simulink model "pid_control_V1"  (R2025b)
settings: Solver=FixedStepAuto  StartTime=0.0  StopTime=tsim  FixedStep=0.01  RelTol=1e-3
undefined symbols (not defined in the file): Cp, F, h_sp, Kd_h, Kd_pitch, Ki_h, Ki_pitch, Kp_h, Kp_pitch, Light, MIL, state, theta_sp, Tp, u_nom, x0
libraries: aerolibactuator x5, ros2lib x2, slpidlib x2, robotcorelib x1, aerolibwind2 x1
settings Model: Creator=sofij  LastModifiedBy=facyu
settings SolverCC: AlgebraicLoopSolver=TrustRegion
settings OptimizationCC: DefaultParameterBehavior=Inlined  EnhancedBackFolding=on  PassReuseOutputArgsAs=Individual arguments  ZeroExternalMemoryAtStartup=off  ZeroInternalMemoryAtStartup=off  MaxStackSize=64  OptimizeBlockOrder=speed  DifferentSizesBufferReuse=on  OptimizationCustomize=off  EfficientTunableParamExpr=on
settings DebuggingCC: ParameterTunabilityLossMsg=error  UnconnectedInputMsg=warning  UnconnectedOutputMsg=warning  UnconnectedLineMsg=warning  SFUnexpectedBacktrackingDiag=warning  SFNoUnconditionalDefaultTransitionDiag=warning
settings HardwareCC: ProdBitPerLong=64.0  ProdHWDeviceType=Intel->x86-64 (Linux 64)  UseEmbeddedCoderFeatures=off
settings ModelReferenceCC: EnableRefExpFcnMdlSchedulingChecks=on
settings SFSimCC: MATLABDynamicMemAlloc=off
settings RTWCC: SystemTargetFile=ert.tlc  HardwareBoard=Robot Operating System 2 (ROS 2)  TLCOptions="-aInlineSetEventsForThisBaseRateFcn=TLC_FALSE -aSuppressMultiTaskScheduler=TLC_FALSE  -aRateBasedStepFcn=0"  TemplateMakefile=ert_default_tmf  GenerateReport=on  Toolchain=Colcon Tools  BuildConfiguration=Debug  LaunchReport=on  TargetLang=C++  GPUComputeCapability=3.5  DLArmComputeVersion=19.05  Description=Embedded Coder
settings CodeAppCC: ForceParamTrailComments=on  IgnoreCustomStorageClasses=off  OperatorAnnotations=on  SimulinkDataObjDesc=on  SFDataObjDesc=on  InsertBlockDesc=on  EnableCustomComments=on
settings ERTTargetCC: ExtModeTransport=2.0  ExtModeStaticAlloc=on  ExtModeAutomaticAllocSize=off  ExtModeMexFile=ext_xcp  ExtModeIntrfLevel=Level2 - Open  RootIOFormat=Structure reference  CodeInterfacePackaging=C++ class  SupportNonInlinedSFcns=on

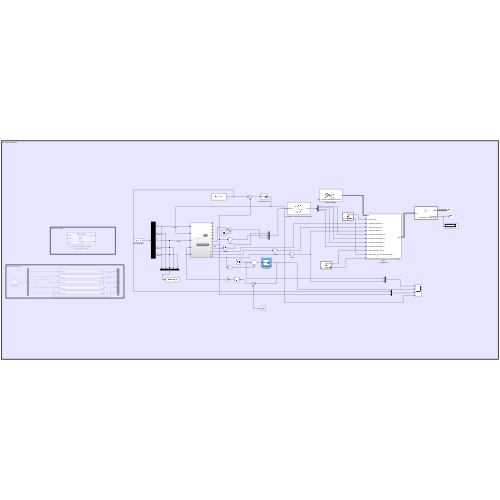
[thumbnail: Simulink's stored preview of the top-level diagram]
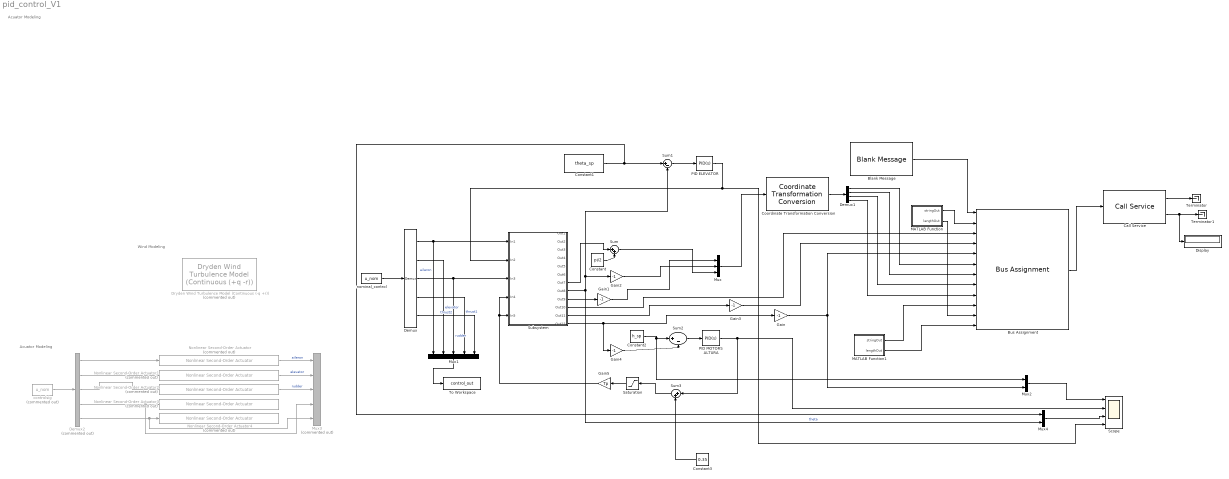
== system pid_control_V1 ==
  note: Wind Modeling
  note: Acuator Modeling
  note: Acuator Modeling
  Blank Message : ros2lib/Blank Message  messageClass=Service Request  entityType=gazebo_msgs/SetEntityState  messageType=gazebo_msgs/SetEntityStateRequest  SampleTime=0.01
  Bus Assignment : BusAssignment  AssignedSignals=state.name,state.pose.position.x,state.pose.position.y,state.pose.position.z,state.pose.orientation.w,state.pose.orientation.z,state.pose.orientation.y,state.pose.orientation.x,state.reference_frame,state.name_SL_Info.CurrentLength,state.reference_frame_SL_Info.CurrentLength
  Call Service : ros2lib/Call Service  topicSource=Specify your own  service=/gazebo/set_entity_state  serviceType=gazebo_msgs/SetEntityState  connectionTimeout=5  ShowErrorCodeOutput=on  legacyBusStruct=off  QOSHistory=Keep last  QOSDepth=1  QOSReliability=Reliable  QOSDurability=Volatile  QOSDeadline=Inf  QOSLifespan=Inf  QOSLiveliness=Automatic  QOSLeaseDuration=Inf  QOSAvoidROSNamespaceConventions=off
  Constant : Constant  Value=pi/2
  Constant1 : Constant  Value=theta_sp
  Constant2 : Constant  Value=h_sp
  Constant3 : Constant  Value=0.35
  Coordinate Transformation Conversion : robotcorelib/Coordinate Transformation Conversion  InputRepresentation=Euler Angles  InputEulerSequence=ZYX  ShowTrVecInputPort=on  OutputRepresentation=Quaternion  OutputEulerSequence=ZYX  ShowTrVecOutputPort=on  SimulateUsing=Interpreted execution
      settings: LibrarySourceBlock=roslib/Utilities/Coordinate Transformation Conversion
  Demux : Demux  Outputs=5
  Demux1 : Demux
  Demux2 : Demux  Commented=on  Outputs=5
  Display : Display
  Dryden Wind Turbulence Model (Continuous (-q +r)) : aerolibwind2/Dryden Wind Turbulence Model  (Continuous (+q -r))  Commented=on  units=Metric (MKS)  spec=MIL-F-8785C  model=Continuous Dryden (-q +r)  W20=15  Wdeg=0  TurbProb=10^-2 - Light  L_high=533.4  Wingspan=10  ts=0.1  Seed=[23341 23342 23343 23344]  T_on=on
  Gain{,1..4} (5 alike) : Gain  Gain=-1
  Gain5 : Gain  Gain=Tp
  MATLAB Function : MATLAB Function  TreatAsAtomicUnit=on
  MATLAB Function1 : MATLAB Function  TreatAsAtomicUnit=on
  Mux : Mux  Inputs=3
  Mux1 : Mux  Inputs=5
  Mux2 : Mux  Inputs=2
  Mux3 : Mux  Commented=on  Inputs=5
  Mux4 : Mux  Inputs=2
  Nonlinear Second-Order Actuator : aerolibactuator/Nonlinear Second-Order Actuator  Commented=on  wn_fin=1  z_fin=0.3  fin_max=15*pi/180  fin_min=-20*pi/180  fin_maxrate=500*pi/180  fin_act_0=0  fin_act_vel=0
  Nonlinear Second-Order Actuator1 : aerolibactuator/Nonlinear Second-Order Actuator  Commented=on  wn_fin=1  z_fin=0.3  fin_max=20*pi/180  fin_min=-20*pi/180  fin_maxrate=500*pi/180  fin_act_0=0  fin_act_vel=0
  Nonlinear Second-Order Actuator2 : aerolibactuator/Nonlinear Second-Order Actuator  Commented=on  wn_fin=1  z_fin=0.3  fin_max=15*pi/180  fin_min=-15*pi/180  fin_maxrate=500*pi/180  fin_act_0=0  fin_act_vel=0
  Nonlinear Second-Order Actuator3 : aerolibactuator/Nonlinear Second-Order Actuator  Commented=on  wn_fin=1  z_fin=0.3  fin_max=100  fin_min=0  fin_maxrate=500*pi/180  fin_act_0=0  fin_act_vel=0
  Nonlinear Second-Order Actuator4 : aerolibactuator/Nonlinear Second-Order Actuator  Commented=on  wn_fin=1  z_fin=0.3  fin_max=100  fin_min=0  fin_maxrate=500*pi/180  fin_act_0=0  fin_act_vel=0
  PID ELEVATOR : slpidlib/PID Controller  Controller=PID  Form=Parallel  TimeDomain=Continuous-time  UseExternalTs=off  SampleTime=-1  IntegratorMethod=Forward Euler  FilterMethod=Forward Euler  ControllerParametersSource=internal  P=Kp_pitch  I=Ki_pitch  UseKiTs=off  D=Kd_pitch  UseExternalDerivativeSource=off  N=100  UseFilter=on  TunerSelectOption=Transfer Function Based (PID Tuner App)  InitialConditionSource=internal  InitialConditionForIntegrator=0  InitialConditionForFilter=0  DifferentiatorICPrevScaledInput=0  ExternalReset=none  TrackingMode=off  Kt=1  LimitOutput=on  SatLimitsSource=internal  UpperSaturationLimit=20*pi/180  LowerSaturationLimit=-20*pi/180  LinearizeAsGain=on  AntiWindupMode=clamping  Kb=1  LimitIntegrator=off  UpperIntegratorSaturationLimit=inf  LowerIntegratorSaturationLimit=-inf  POutMin=[]  POutMax=[]  IOutMin=[]  IOutMax=[]  DOutMin=[]  DOutMax=[]  NOutMin=[]  NOutMax=[]  SumOutMin=[]  SumOutMax=[]  SaturationOutMin=[]  SaturationOutMax=[]  PParamMin=[]  PParamMax=[]  IParamMin=[]  IParamMax=[]  DParamMin=[]  DParamMax=[]  NParamMin=[]  NParamMax=[]  KbParamMin=[]  KbParamMax=[]  KtParamMin=[]  KtParamMax=[]  KbOutMin=[]  KbOutMax=[]  KtOutMin=[]  KtOutMax=[]  IntegratorOutMin=[]  IntegratorOutMax=[]  FilterOutMin=[]  FilterOutMax=[]  SumI1OutMin=[]  SumI1OutMax=[]  SumI2OutMin=[]  SumI2OutMax=[]  SumI3OutMin=[]  SumI3OutMax=[]  SumI4OutMin=[]  SumI4OutMax=[]  SumDOutMin=[]  SumDOutMax=[]  DifferentiatorOutMin=[]  DifferentiatorOutMax=[]  FilterDiffOutCoefMin=[]  FilterDiffOutCoefMax=[]  ReciprocalOutMin=[]  ReciprocalOutMax=[]  SumDenOutMin=[]  SumDenOutMax=[]  SumNumOutMin=[]  SumNumOutMax=[]  DivideOutMin=[]  DivideOutMax=[]  UdiffTsProdOutMin=[]  UdiffTsProdOutMax=[]  NTsProdOutMin=[]  NTsProdOutMax=[]  UintegralTsProdOutMin=[]  UintegralTsProdOutMax=[]  UngainTsProdOutMin=[]  UngainTsProdOutMax=[]  ClampingZeroOutDataTypeStr=Inherit: Inherit via back propagation  ClampingZeroOutMin=[]  ClampingZeroOutMax=[]  FilterDenConstantOutDataTypeStr=Inherit: Inherit via back propagation  FilterDenConstantOutMin=[]  FilterDenConstantOutMax=[]  PCopyOutDataTypeStr=Inherit: Inherit via back propagation  PCopyOutMin=[]  PCopyOutMax=[]  NCopyOutDataTypeStr=Inherit: Inherit via back propagation  NCopyOutMin=[]  NCopyOutMax=[]  IntegratorContinuousStateAttributes=''  IntegratorStateMustResolveToSignalObject=off  IntegratorRTWStateStorageClass=Auto  FilterContinuousStateAttributes=''  FilterStateMustResolveToSignalObject=off  FilterRTWStateStorageClass=Auto  ParallelPVariant=InternalParameters  IdealPVariant=Disabled  IVariant=InternalParameters  DVariant=InternalParameters  IntegratorVariant=Continuous  SatVariant=Enabled  AWVariant=ContClampingParallel  PCopyVariant=Disabled  TRVariant=Disabled  FdbkBlocksVariant=Forward  IdealPFdbkVariant=Disabled  SatFdbkVariant=Disabled  DerivativeFilterVariant=ContFilter  NVariant=InternalParameters  NCopyVariant=Disabled  FilterICVariant=InternalICsFilter  IntegratorICVariant=InternalICs  ExternalResetVariant=Disabled  TRSumVariant=Passthrough  SumFdbkVariant=Disabled  SumVariant=Sum_PID  TsampFilterVariant=InternalTs  TsampNgainVariant=Passthrough  TsampIntegralVariant=Disabled_SignalSpec  ExternalSaturationOutDataTypeStr=Inherit: Same as second input  DerivativeSourceVariant=ErrorSignal  PreIntVariant=InternalPreInt
  PID MOTORS ALTURA : slpidlib/PID Controller  Controller=PID  Form=Parallel  TimeDomain=Continuous-time  UseExternalTs=off  SampleTime=-1  IntegratorMethod=Forward Euler  FilterMethod=Forward Euler  ControllerParametersSource=internal  P=Kp_h  I=Ki_h  UseKiTs=off  D=Kd_h  UseExternalDerivativeSource=off  N=100  UseFilter=on  TunerSelectOption=Transfer Function Based (PID Tuner App)  InitialConditionSource=internal  InitialConditionForIntegrator=0.3  InitialConditionForFilter=0  DifferentiatorICPrevScaledInput=0  ExternalReset=none  TrackingMode=off  Kt=1  LimitOutput=on  SatLimitsSource=internal  UpperSaturationLimit=1  LowerSaturationLimit=0  LinearizeAsGain=on  AntiWindupMode=clamping  Kb=1  LimitIntegrator=off  UpperIntegratorSaturationLimit=inf  LowerIntegratorSaturationLimit=-inf  POutMin=[]  POutMax=[]  IOutMin=[]  IOutMax=[]  DOutMin=[]  DOutMax=[]  NOutMin=[]  NOutMax=[]  SumOutMin=[]  SumOutMax=[]  SaturationOutMin=[]  SaturationOutMax=[]  PParamMin=[]  PParamMax=[]  IParamMin=[]  IParamMax=[]  DParamMin=[]  DParamMax=[]  NParamMin=[]  NParamMax=[]  KbParamMin=[]  KbParamMax=[]  KtParamMin=[]  KtParamMax=[]  KbOutMin=[]  KbOutMax=[]  KtOutMin=[]  KtOutMax=[]  IntegratorOutMin=[]  IntegratorOutMax=[]  FilterOutMin=[]  FilterOutMax=[]  SumI1OutMin=[]  SumI1OutMax=[]  SumI2OutMin=[]  SumI2OutMax=[]  SumI3OutMin=[]  SumI3OutMax=[]  SumI4OutMin=[]  SumI4OutMax=[]  SumDOutMin=[]  SumDOutMax=[]  DifferentiatorOutMin=[]  DifferentiatorOutMax=[]  FilterDiffOutCoefMin=[]  FilterDiffOutCoefMax=[]  ReciprocalOutMin=[]  ReciprocalOutMax=[]  SumDenOutMin=[]  SumDenOutMax=[]  SumNumOutMin=[]  SumNumOutMax=[]  DivideOutMin=[]  DivideOutMax=[]  UdiffTsProdOutMin=[]  UdiffTsProdOutMax=[]  NTsProdOutMin=[]  NTsProdOutMax=[]  UintegralTsProdOutMin=[]  UintegralTsProdOutMax=[]  UngainTsProdOutMin=[]  UngainTsProdOutMax=[]  ClampingZeroOutDataTypeStr=Inherit: Inherit via back propagation  ClampingZeroOutMin=[]  ClampingZeroOutMax=[]  FilterDenConstantOutDataTypeStr=Inherit: Inherit via back propagation  FilterDenConstantOutMin=[]  FilterDenConstantOutMax=[]  PCopyOutDataTypeStr=Inherit: Inherit via back propagation  PCopyOutMin=[]  PCopyOutMax=[]  NCopyOutDataTypeStr=Inherit: Inherit via back propagation  NCopyOutMin=[]  NCopyOutMax=[]  IntegratorContinuousStateAttributes=''  IntegratorStateMustResolveToSignalObject=off  IntegratorRTWStateStorageClass=Auto  FilterContinuousStateAttributes=''  FilterStateMustResolveToSignalObject=off  FilterRTWStateStorageClass=Auto  ParallelPVariant=InternalParameters  IdealPVariant=Disabled  IVariant=InternalParameters  DVariant=InternalParameters  IntegratorVariant=Continuous  SatVariant=Enabled  AWVariant=ContClampingParallel  PCopyVariant=Disabled  TRVariant=Disabled  FdbkBlocksVariant=Forward  IdealPFdbkVariant=Disabled  SatFdbkVariant=Disabled  DerivativeFilterVariant=ContFilter  NVariant=InternalParameters  NCopyVariant=Disabled  FilterICVariant=InternalICsFilter  IntegratorICVariant=InternalICs  ExternalResetVariant=Disabled  TRSumVariant=Passthrough  SumFdbkVariant=Disabled  SumVariant=Sum_PID  TsampFilterVariant=InternalTs  TsampNgainVariant=Passthrough  TsampIntegralVariant=Disabled_SignalSpec  ExternalSaturationOutDataTypeStr=Inherit: Same as second input  DerivativeSourceVariant=ErrorSignal  PreIntVariant=InternalPreInt
  Saturation : Saturate  UpperLimit=1.0  LowerLimit=0.3
  Scope : Scope  NumInputPorts=4
      settings: ActiveDisplayYMinimum=-1.7310534077448412  ActiveDisplayYMaximum=4.7021232527921839  DataLoggingVariableName=ScopeData4
  Subsystem : Subsystem
  Sum : Sum  Inputs=|++
  Sum1 : Sum  Inputs=|+-
  Sum2 : Sum  Inputs=|+-
  Sum3 : Sum  Inputs=|++
  Terminator : Terminator
  Terminator1 : Terminator
  To Workspace : ToWorkspace  VariableName=control_out  SampleTime=-1
      settings: Save2DSignal=2-D array (concatenate along first dimension)
  controlsig : Constant  Commented=on  Value=u_nom
  nominal_control : Constant  Value=u_nom
  wires:
  controlsig/1 -> Demux2/1
  Nonlinear Second-Order Actuator/1 -> Mux3/1  "aileron"
  Demux2/1 -> Nonlinear Second-Order Actuator/1
  Demux2/5 -> Mux3/5, Nonlinear Second-Order Actuator4/1
  Demux2/4 -> Mux3/4, Nonlinear Second-Order Actuator3/1
  Demux2/3 -> Nonlinear Second-Order Actuator2/1
  Demux2/2 -> Nonlinear Second-Order Actuator1/1
  Nonlinear Second-Order Actuator2/1 -> Mux3/3  "rudder"
  Nonlinear Second-Order Actuator1/1 -> Mux3/2  "elevator"
  Demux/3 -> Mux1/3, Subsystem/3(In3)  "rudder"
  nominal_control/1 -> Demux/1
  Demux/1 -> Subsystem/1(In1), Mux1/1  "aileron"
  Blank Message/1 -> Bus Assignment/1
  Subsystem/10(Out10) -> Bus Assignment/3
  Subsystem/11(Out11) -> Gain3/1
  Subsystem/12(Out12) -> Gain4/1, Gain/1
  Subsystem/8(Out8) -> Mux4/2, Gain2/1, Sum1/2  "theta"
  Subsystem/9(Out9) -> Gain1/1
  Mux/1 -> Coordinate Transformation Conversion/1
  Coordinate Transformation Conversion/1 -> Demux1/1
  Demux1/1 -> Bus Assignment/6
  Demux1/2 -> Bus Assignment/7
  Demux1/3 -> Bus Assignment/8
  Demux1/4 -> Bus Assignment/9
  Bus Assignment/1 -> Call Service/1
  Gain/1 -> Mux2/2, Bus Assignment/5
  Call Service/1 -> Terminator/1
  Call Service/2 -> Display/1, Terminator1/1
  MATLAB Function/1(stringOut) -> Bus Assignment/2
  MATLAB Function1/1(stringOut) -> Bus Assignment/10
  MATLAB Function/2(lengthOut) -> Bus Assignment/11
  MATLAB Function1/2(lengthOut) -> Bus Assignment/12
  Gain2/1 -> Mux/2
  Subsystem/7(Out7) -> Sum/1
  Gain3/1 -> Bus Assignment/4
  Gain1/1 -> Mux/1
  Sum/1 -> Mux/3
  Constant/1 -> Sum/2
  Constant1/1 -> Sum1/1, Mux4/1
  Sum1/1 -> PID ELEVATOR/1
  PID ELEVATOR/1 -> Scope/4, Subsystem/2(In2)
  Constant2/1 -> Mux2/1, Sum2/1
  Gain4/1 -> Sum2/2
  Sum2/1 -> PID MOTORS ALTURA/1
  PID MOTORS ALTURA/1 -> Sum3/1, Scope/2
  Mux2/1 -> Scope/1
  Mux4/1 -> Scope/3
  Gain5/1 -> Subsystem/5(In5), Subsystem/4(In4)
  Mux1/1 -> To Workspace/1
  Demux/2 -> Mux1/2  "elevator"
  Demux/4 -> Mux1/4  "thrust1"
  Demux/5 -> Mux1/5  "thrust2"
  Constant3/1 -> Sum3/2
  Saturation/1 -> Gain5/1
  Sum3/1 -> Saturation/1

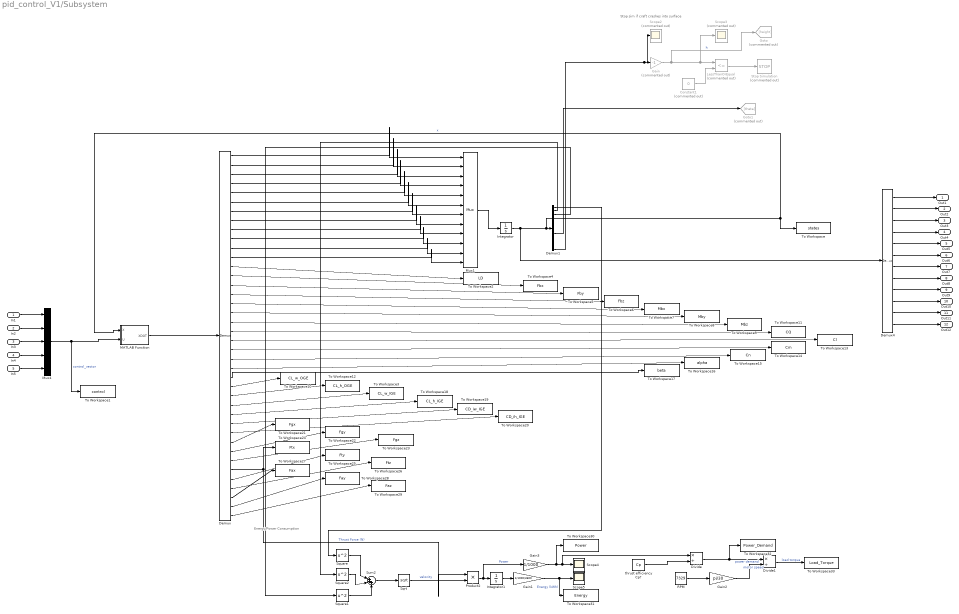
== system pid_control_V1/Subsystem ==
  note: Stop sim if craft crashes into surface
  note: Energy/Power Consumption
  In1 : Inport
  In2 : Inport  Port=2
  In3 : Inport  Port=3
  In4 : Inport  Port=4
  In5 : Inport  Port=5
  Constant1 : Constant  Commented=on  Value=0
  Demux : Demux  Outputs=40
  Demux1 : Demux  Outputs=12
  Demux4 : Demux  Outputs=12
  Divide : Product  Inputs=*/
  Divide1 : Product  Inputs=*/
  Gain : Gain  Commented=on  Gain=-1
  Gain1 : Gain  Gain=1/1000/3600
  Gain2 : Gain  Gain=pi/30
  Gain3 : Gain  Gain=1/1000
  Goto : Goto  Commented=on  GotoTag=height
  Goto1 : Goto  Commented=on  GotoTag=theta
  Integrator : Integrator  InitialCondition=x0
  Integrator1 : Integrator
  LessThanOrEqual : RelationalOperator  Commented=on  Operator=<=  OutDataTypeStr=boolean  RndMeth=Simplest  InputSameDT=off
  MATLAB Function : MATLAB Function  TreatAsAtomicUnit=on
  Mux1 : Mux  Inputs=12
  Mux4 : Mux  Inputs=5
  Product2 : Product
  RPM : Constant  Value=7329
  Scope2 : Scope  Commented=on
      settings: ActiveDisplayYMinimum=-1.36989  ActiveDisplayYMaximum=0.16067
  Scope3 : Scope  Commented=on
      settings: ActiveDisplayYMinimum=-0.16067  ActiveDisplayYMaximum=1.36989  DataLoggingVariableName=ScopeData2
  Scope4 : Scope
      settings: ActiveDisplayYMinimum=-1  ActiveDisplayYMaximum=1  DataLoggingVariableName=ScopeData3
  Scope5 : Scope
  Sqrt : Sqrt
  Square : Math  Operator=square
  Square1 : Math  Operator=square
  Square2 : Math  Operator=square
  Stop Simulation : Stop  Commented=on
  Sum2 : Sum  Inputs=|+++
  To Workspace : ToWorkspace  VariableName=states  SampleTime=-1
  To Workspace1 : ToWorkspace  VariableName=control  SampleTime=-1
  To Workspace10 : ToWorkspace  VariableName=CL_w_OGE  SampleTime=-1
      settings: Save2DSignal=2-D array (concatenate along first dimension)
  To Workspace11 : ToWorkspace  VariableName=CQ  SampleTime=-1
      settings: Save2DSignal=2-D array (concatenate along first dimension)
  To Workspace12 : ToWorkspace  VariableName=CL_h_OGE  SampleTime=-1
      settings: Save2DSignal=2-D array (concatenate along first dimension)
  To Workspace13 : ToWorkspace  VariableName=Cl  SampleTime=-1
      settings: Save2DSignal=2-D array (concatenate along first dimension)
  To Workspace14 : ToWorkspace  VariableName=Cm  SampleTime=-1
      settings: Save2DSignal=2-D array (concatenate along first dimension)
  To Workspace15 : ToWorkspace  VariableName=Cn  SampleTime=-1
      settings: Save2DSignal=2-D array (concatenate along first dimension)
  To Workspace16 : ToWorkspace  VariableName=alpha  SampleTime=-1
      settings: Save2DSignal=2-D array (concatenate along first dimension)
  To Workspace17 : ToWorkspace  VariableName=beta  SampleTime=-1
      settings: Save2DSignal=2-D array (concatenate along first dimension)
  To Workspace18 : ToWorkspace  VariableName=CL_h_IGE  SampleTime=-1
      settings: Save2DSignal=2-D array (concatenate along first dimension)
  To Workspace19 : ToWorkspace  VariableName=CD_iw_IGE  SampleTime=-1
      settings: Save2DSignal=2-D array (concatenate along first dimension)
  To Workspace2 : ToWorkspace  VariableName=LD  SampleTime=-1
      settings: Save2DSignal=2-D array (concatenate along first dimension)
  To Workspace20 : ToWorkspace  VariableName=CD_ih_IGE  SampleTime=-1
      settings: Save2DSignal=2-D array (concatenate along first dimension)
  To Workspace21 : ToWorkspace  VariableName=Fgx  SampleTime=-1
      settings: Save2DSignal=2-D array (concatenate along first dimension)
  To Workspace22 : ToWorkspace  VariableName=Fgy  SampleTime=-1
      settings: Save2DSignal=2-D array (concatenate along first dimension)
  To Workspace23 : ToWorkspace  VariableName=Fgz  SampleTime=-1
      settings: Save2DSignal=2-D array (concatenate along first dimension)
  To Workspace24 : ToWorkspace  VariableName=Ftx  SampleTime=-1
      settings: Save2DSignal=2-D array (concatenate along first dimension)
  To Workspace25 : ToWorkspace  VariableName=Fty  SampleTime=-1
      settings: Save2DSignal=2-D array (concatenate along first dimension)
  To Workspace26 : ToWorkspace  VariableName=Ftz  SampleTime=-1
      settings: Save2DSignal=2-D array (concatenate along first dimension)
  To Workspace27 : ToWorkspace  VariableName=Fax  SampleTime=-1
      settings: Save2DSignal=2-D array (concatenate along first dimension)
  To Workspace28 : ToWorkspace  VariableName=Fay  SampleTime=-1
      settings: Save2DSignal=2-D array (concatenate along first dimension)
  To Workspace29 : ToWorkspace  VariableName=Faz  SampleTime=-1
      settings: Save2DSignal=2-D array (concatenate along first dimension)
  To Workspace3 : ToWorkspace  VariableName=CL_w_IGE  SampleTime=-1
      settings: Save2DSignal=2-D array (concatenate along first dimension)
  To Workspace30 : ToWorkspace  VariableName=Power  SampleTime=-1
      settings: Save2DSignal=2-D array (concatenate along first dimension)
  To Workspace31 : ToWorkspace  VariableName=Energy  SampleTime=-1
      settings: Save2DSignal=2-D array (concatenate along first dimension)
  To Workspace32 : ToWorkspace  VariableName=Power_Demand  SampleTime=-1
      settings: Save2DSignal=2-D array (concatenate along first dimension)
  To Workspace33 : ToWorkspace  VariableName=Load_Torque  SampleTime=-1
      settings: Save2DSignal=2-D array (concatenate along first dimension)
  To Workspace4 : ToWorkspace  VariableName=Fbx  SampleTime=-1
      settings: Save2DSignal=2-D array (concatenate along first dimension)
  To Workspace5 : ToWorkspace  VariableName=Fby  SampleTime=-1
      settings: Save2DSignal=2-D array (concatenate along first dimension)
  To Workspace6 : ToWorkspace  VariableName=Fbz  SampleTime=-1
      settings: Save2DSignal=2-D array (concatenate along first dimension)
  To Workspace7 : ToWorkspace  VariableName=Mbx  SampleTime=-1
      settings: Save2DSignal=2-D array (concatenate along first dimension)
  To Workspace8 : ToWorkspace  VariableName=Mby  SampleTime=-1
      settings: Save2DSignal=2-D array (concatenate along first dimension)
  To Workspace9 : ToWorkspace  VariableName=Mbz  SampleTime=-1
      settings: Save2DSignal=2-D array (concatenate along first dimension)
  thrust efficiency Cp? : Constant  Value=Cp
  Out1 : Outport
  Out2 : Outport  Port=2
  Out3 : Outport  Port=3
  Out4 : Outport  Port=4
  Out5 : Outport  Port=5
  Out6 : Outport  Port=6
  Out7 : Outport  Port=7
  Out8 : Outport  Port=8
  Out9 : Outport  Port=9
  Out10 : Outport  Port=10
  Out11 : Outport  Port=11
  Out12 : Outport  Port=12
  wires:
  Demux4/3 -> Out3/1
  Mux4/1 -> MATLAB Function/2(U), To Workspace1/1  "control_vector"
  In1/1 -> Mux4/1
  Product2/1 -> Gain3/1, Integrator1/1  "Power"
  Demux/27 -> To Workspace12/1
  Demux/31 -> To Workspace20/1
  Demux/4 -> Mux1/4
  Demux/33 -> To Workspace22/1
  Demux1/8 -> Goto1/1
  Divide/1 -> To Workspace32/1, Divide1/1  "power demand"
  Gain1/1 -> To Workspace31/1, Scope5/1  "Energy (kWh)"
  Demux1/2 -> Square2/1
  Demux/8 -> Mux1/8
  LessThanOrEqual/1 -> Stop Simulation/1
  RPM/1 -> Gain2/1
  Demux/2 -> Mux1/2
  Demux/21 -> To Workspace13/1
  Demux/29 -> To Workspace18/1
  Demux/22 -> To Workspace14/1
  Demux/36 -> To Workspace25/1
  Demux/38 -> To Workspace27/1
  Demux/40 -> To Workspace29/1
  Demux/28 -> To Workspace3/1
  Demux/17 -> To Workspace7/1
  Gain3/1 -> To Workspace30/1, Divide/1, Scope4/1
  Demux1/3 -> Square1/1
  Demux/18 -> To Workspace8/1
  Divide1/1 -> To Workspace33/1  "load torque"
  Constant1/1 -> LessThanOrEqual/2
  Sqrt/1 -> Product2/2  "velocity"
  Square2/1 -> Sum2/2
  Square1/1 -> Sum2/3
  Demux/39 -> To Workspace28/1
  Gain2/1 -> Divide1/2  "motor speed"
  Demux/25 -> To Workspace17/1
  Demux/23 -> To Workspace15/1
  Demux/9 -> Mux1/9
  Demux1/1 -> Square/1
  Demux/26 -> To Workspace10/1
  Square/1 -> Sum2/1
  thrust efficiency Cp?/1 -> Divide/2
  Demux/14 -> To Workspace4/1
  Demux/15 -> To Workspace5/1
  Sum2/1 -> Sqrt/1
  Demux/11 -> Mux1/11
  Demux/37 -> To Workspace26/1
  Demux/19 -> To Workspace9/1
  Gain/1 -> Goto/1, Scope3/1, LessThanOrEqual/1  "h"
  Demux/20 -> To Workspace11/1
  Demux/7 -> Mux1/7
  Demux/3 -> Mux1/3
  MATLAB Function/1(XDOT) -> Demux/1
  Demux/35 -> Product2/1, To Workspace24/1  "Thrust Force (N)"
  Integrator/1 -> Demux4/1, To Workspace/1, MATLAB Function/1(X), Demux1/1  "x"
  Demux/24 -> To Workspace16/1
  Demux/6 -> Mux1/6
  Demux/5 -> Mux1/5
  Mux1/1 -> Integrator/1
  Demux/30 -> To Workspace19/1
  In5/1 -> Mux4/5
  In4/1 -> Mux4/4
  Demux/1 -> Mux1/1
  In2/1 -> Mux4/2
  Demux/10 -> Mux1/10
  Demux4/11 -> Out11/1
  Demux4/6 -> Out6/1
  Demux/13 -> To Workspace2/1
  Demux4/2 -> Out2/1
  Demux4/9 -> Out9/1
  Demux4/1 -> Out1/1
  Integrator1/1 -> Gain1/1
  Demux4/4 -> Out4/1
  Demux/34 -> To Workspace23/1
  Demux4/10 -> Out10/1
  Demux4/8 -> Out8/1
  Demux/12 -> Mux1/12
  Demux/16 -> To Workspace6/1
  Demux/32 -> To Workspace21/1
  Demux4/5 -> Out5/1
  Demux1/12 -> Scope2/1, Gain/1
  In3/1 -> Mux4/3
  Demux4/7 -> Out7/1
  Demux4/12 -> Out12/1

== matlab function pid_control_V1/Subsystem/MATLAB Function ==
  data: X input; XDOT output; U input
function XDOT  = Model(X,U)
%#codegen
%-----------STATE AND CONTROL VECTORS-------------
x1=X(1); x2=X(2); x3=X(3); x4=X(4); x5=X(5); x6=X(6);
x7=X(7); x8=X(8); x9=X(9); x10=X(10); x11=X(11); x12=X(12);

u1=U(1); u2=U(2); u3=U(3); u4=U(4); u5=U(5);

%-----------SYSTEM PARAMETERS------------------------------
m = 112; % Ajustado al original para poder volar
bw = 5.02; bh = 2.74; cbar = 0.646; 
Sw = 3.334; Sh = 1.128; 
ARw = 7.5; ARh = 6.7; TRw = 0.4; TRh = 0.5;

Xcg = 0; Ycg = 0; Zcg = 0;
Xac = 0.097; Yac = 0; Zac = -0.06;
Xapt1 = -0.519; Yapt1 = 0.6; Zapt1 = 0.285;
Xapt2 = -0.519; Yapt2 = -0.6; Zapt2 = 0.285;

rho = 1.225; g = 9.81;
e0w = 0.9; e0h = 0.9;
alpha_0w = -3.75*pi/180; alpha_0h = -4.25*pi/180;
iw = 2.5*pi/180; % Incidencia moderada para no dispararse
ih = 1.5*pi/180; 
eps = 0; zw = 0.363; zh = 0.72; CD_0 = 0.0306;
Tp = 0.125*10^(-3);

% Saturación
u1 = max(min(u1, 15*pi/180), -20*pi/180);
u2 = max(min(u2, 20*pi/180), -20*pi/180);
u3 = max(min(u3, 15*pi/180), -15*pi/180);
u4 = max(min(u4, Tp), 0);
u5 = max(min(u5, Tp), 0);

% VARIABLES INTERMEDIAS
phi=x7; theta=x8; psi=x9;
Rb_v = [cos(theta)*cos(psi), cos(theta)*sin(psi), -sin(theta);
        sin(phi)*sin(theta)*cos(psi)-cos(phi)*sin(psi), sin(phi)*sin(theta)*sin(psi)+cos(phi)*cos(psi), sin(phi)*cos(theta);
        cos(phi)*sin(theta)*cos(psi)+sin(phi)*sin(psi), cos(phi)*sin(theta)*sin(psi)-sin(phi)*cos(psi), cos(phi)*cos(theta)];

Va = sqrt(x1^2+x2^2+x3^2);
if Va == 0, Va = 0.001; end % Evitar NaN en inicio
alpha = atan2(x3,x1);
beta = asin(x2/Va);

h = -x12;
hw = max(0.001, h-zw); 
hh = h+zh;
Q = 0.5*rho*Va^2;

wbe_b = [x4;x5;x6];
V_b = [x1;x2;x3];

% Aerodinámica
mu_Lw = 1 + (1 - 2.25*(TRw^0.00273 - 0.997)*((ARw^0.717)+13.6))*(288*abs(hw/bw)^0.787*exp(-9.14*(abs(hw/bw)^0.327)))/(ARw^0.882);
mu_Lh = 1 + (1 - 2.25*(TRh^0.00273 - 0.997)*((ARh^0.717)+13.6))*(288*abs(hh/bh)^0.787*exp(-9.14*(abs(hh/bh)^0.327)))/(ARh^0.882);

C_L_e = -0.00141*u2^2+0.0307*u2;
CL_w_OGE = 2*pi*(ARw/(ARw+2))*(alpha-alpha_0w+iw);
CL_h_OGE = 2*pi*(ARh/(ARh+2))*(alpha-alpha_0h+ih+eps);

CL_w_IGE = CL_w_OGE*mu_Lw;
CL_h_IGE = (CL_h_OGE + C_L_e)*mu_Lh;

mu_Dw = 1 - exp(-10.1*(abs(hw/bw)^0.686));
mu_Dh = 1 - exp(-10.1*(abs(hh/bh)^0.686));

CD_iw_IGE = (CL_w_OGE^2)/(pi*ARw*e0w)*mu_Dw;
CD_ih_IGE = (CL_h_OGE^2)/(pi*ARh*e0h)*mu_Dh;
C_D_e = -0.0000108*u2^2+0.000715*u2;

Dtot = Q*(CD_0*Sw + CD_iw_IGE*Sw + CD_ih_IGE*Sh + C_D_e*Sh);
Ltot = Q*(CL_w_IGE*Sw + CL_h_IGE*Sh);
CQ = -0.019*beta*180/pi;

FA_s = [-Dtot; CQ*Q*Sw; -Ltot];
C_bs = [cos(alpha) 0 -sin(alpha); 0 1 0; sin(alpha) 0 cos(alpha)];
FA_b = C_bs*FA_s;

Cm_alpha = -1.14; Cm_q = -5.0; Cm_de = -3.0; Cm_h = 0.05;
Delta_Cm_IGE = -Cm_h * exp(-4.0 * abs(hw/bw));
Cl = -0.0005*beta*180/pi;
Cm = Cm_alpha*alpha + Delta_Cm_IGE + Cm_q*(x5*cbar/(2*Va)) + Cm_de*u2; 
Cn = -0.002*beta*180/pi;

MAcg_b = [Cl;Cm;Cn].*[bw*Q*Sw; cbar*Q*Sw; bw*Q*Sw];

% Motores (Corregido empuje en Z)
km = 37.42; Cp = 0.57; D = 0.635; Sp = pi*(D^2/4);
Vd1 = Va + (u4/Tp)*(km-Va); Tp1 = 0.5*rho*Sp*Cp*Vd1*(Vd1-Va);
Vd2 = Va + (u5/Tp)*(km-Va); Tp2 = 0.5*rho*Sp*Cp*Vd2*(Vd2-Va);

FE1_b = [Tp1*cos(-5*pi/180); 0; Tp1*sin(5*pi/180)];
FE2_b = [Tp2*cos(-5*pi/180); 0; Tp2*sin(5*pi/180)];
FE_b = FE1_b + FE2_b;

MEcg1_b = cross([Xcg-Xapt1; Yapt1-Ycg; Zcg-Zapt1], FE1_b);
MEcg2_b = cross([Xcg-Xapt2; Yapt2-Ycg; Zcg-Zapt2], FE2_b);
MEcg_b = MEcg1_b + MEcg2_b;

g_b = [-g*sin(theta); g*cos(theta)*sin(phi); g*cos(theta)*cos(phi)];
Fg_b = m*g_b;

% Inercia
Ib = [39.71 0 8.97; 0 85.51 0; 8.97 0 114.39];
invIb = inv(Ib);

F_b = Fg_b + FE_b + FA_b;
x1to3dot = (1/m)*F_b - cross(wbe_b,V_b);

Mcg_b = MAcg_b + MEcg_b;
x4to6dot = invIb*(Mcg_b - cross(wbe_b,Ib*wbe_b));

H_phi = [1 sin(phi)*tan(theta) cos(phi)*tan(theta);
         0 cos(phi) -sin(phi);
         0 sin(phi)/cos(theta) cos(phi)/cos(theta)];
x7to9dot = H_phi*wbe_b;
x10to12dot = rot_body_to_ned(X); % Llamada a la cinemática

XDOT = [x1to3dot; x4to6dot; x7to9dot; x10to12dot; 0; F_b; Mcg_b; CQ; Cl; Cm; Cn; alpha; beta; CL_w_OGE; CL_h_OGE; CL_w_IGE; CL_h_IGE; CD_iw_IGE; CD_ih_IGE; Fg_b; FE_b; FA_b];
end

%------------------------- LOCAL FUNCTIONS -------------------------
function [V_NED] = rot_body_to_ned(X)
%#codegen
V_body=[X(1);X(2);X(3)];

roll  = X(7); % phi
pitch = X(8); % theta
yaw   = X(9); % psi

R = [cos(pitch)*cos(yaw), sin(roll)*sin(pitch)*cos(yaw)-cos(roll)*sin(yaw), cos(roll)*sin(pitch)*cos(yaw)+sin(roll)*sin(yaw);
     cos(pitch)*sin(yaw), sin(roll)*sin(pitch)*sin(yaw)+cos(roll)*cos(yaw), cos(roll)*sin(pitch)*sin(yaw)-sin(roll)*cos(yaw);
    -sin(pitch),          sin(roll)*cos(pitch),                             cos(roll)*cos(pitch)];

V_NED = R * V_body;
V_NED = [V_NED(1); V_NED(2); V_NED(3)];
end

== matlab function pid_control_V1/MATLAB Function1 ==
  data: stringOut output; lengthOut output
function [stringOut, lengthOut] = frameToROS()

    % Define el marco de referencia
    miTexto = 'world';
    
    % Crea el vector columna de 128 ceros tipo uint8
    stringOut = zeros(128, 1, 'uint8');
    
    % Copia las letras de 'world' al inicio
    stringOut(1:length(miTexto)) = uint8(miTexto);
    
    % Calcula la longitud exacta para ROS 2
    lengthOut = uint32(length(miTexto));

end

== matlab function pid_control_V1/MATLAB Function ==
  data: stringOut output; lengthOut output
function [stringOut, lengthOut] = stringToROS()
    
    % Define la palabra exacta (fíjate que sea el mismo nombre que en el .world)
    miTexto = 'ekranoplano';
    
    % Crea el vector de 128 posiciones
    stringOut = zeros(128, 1, 'uint8');
    stringOut(1:length(miTexto)) = uint8(miTexto);
    
    % Calcula la longitud para ROS (en tipo uint32)
    lengthOut = uint32(length(miTexto));
    
end
